simulink model "Coupled_GP_fit"  (R2018b)
settings: Solver=FixedStepAuto  StartTime=0.0  StopTime=t_end  FixedStep=ts  MinStep=1/1e5  RelTol=1e-3
values from neighbouring files (symbols this model uses):
  a0 = omega_n^3    (= 248050213.442)    [TwoLink_init.m]    (also in init.m = 31006276.6803)
  a1 = 3*omega_n^2    (= 1184352.52813)    [TwoLink_init.m]    (also in init.m = 296088.132033)
  a2 = 3*omega_n    (= 1884.95559215)    [TwoLink_init.m]    (also in init.m = 942.477796077)
  b1 = b(:,1)    [init.m]
  b2 = b(:,2)    [init.m]
  D = 50    [Train_SSGP.m]    (also in init.m = 21)
  g = 9.81    [init.m]
  h = 1    [init.m]
  I_limit = 2000    [TwoLink_init.m]
  L1 = 1    [init.m]
  L2 = 1    [init.m]
  m1 = 1    [init.m]
  m2 = 5    [init.m]
  mu_X = mean(xTrain')    [Train_SSGP.m]    (also in init.m = zeros(1,size(n,2)))
  mu_Y = mean(yTrain')    [Train_SSGP.m]    (also in init.m = zeros(1,size(Q,2)))
  N = size(xTrain,2)    [Train_SSGP.m]    (also in init.m = length(noiseSignal))
  r = 5e3    (= 5000)    [init.m]
  R1 = squeeze(R(1,:,:))    [init.m]
  R2 = squeeze(R(2,:,:))    [init.m]
  s = xTrain(:,i_s)'    [Train_SSGP.m]    (also in TwoLink_init.m = tf('s'))
  seed = randi(1e6)    [init.m]
  sf1 = sf(1)    [init.m]
  sf2 = sf(2)    [init.m]
  sig_X = std(xTrain')    [Train_SSGP.m]    (also in init.m = ones(1,size(n,2)))
  sig_Y = std(yTrain')    [Train_SSGP.m]    (also in init.m = ones(1,size(n,2)))
  SIGMA1 = squeeze(SIGMA(1,:,:))    [init.m]
  SIGMA2 = squeeze(SIGMA(2,:,:))    [init.m]
  sp_ts = 2.5    [init.m]
  t_learn = 0    [init.m]
  t_predict = 50    [init.m]
  tm = 2    [init.m]
  ts = 1/1000    (= 0.001)    [Train_SSGP.m]    (also in TwoLink_init.m; init.m)
  w1 = w(:,1)    [init.m]
  w2 = w(:,2)    [init.m]
  X = squeeze(xTraining(:,1,:))'    [init.m]    (also in plot_train_data.m = squeeze(input_vector.Data(:,:,ts_index)))
  Y = yTraining    [init.m]
undefined symbols (not defined in the file or in its folder): DiscIntNeverNeededParam, FF, noise, PID, Z
libraries: sm_lib x13, simulink x6, nesl_utility x5
(part 2 of 2)

== system Coupled_GP_fit/Setpoint Generator/TDfhan1 ==
  V : Inport
  Constant : Constant  Value=r
  Constant1 : Constant  Value=h
  Discrete-Time Integrator : DiscreteIntegrator  gainval=1  SampleTime=ts  ICPrevOutput=DiscIntNeverNeededParam  ICPrevScaledInput=DiscIntNeverNeededParam
  Discrete-Time Integrator1 : DiscreteIntegrator  gainval=1  SampleTime=ts  ICPrevOutput=DiscIntNeverNeededParam  ICPrevScaledInput=DiscIntNeverNeededParam
  MATLAB Function2 : MATLAB Function  TreatAsAtomicUnit=on
  Scope : Scope  NumInputPorts=3
  Sum : Sum  Inputs=+-|
  V1 : Outport
  V2 : Outport  Port=2
  V3 : Outport  Port=3
  wires:
  Discrete-Time Integrator/1 -> Discrete-Time Integrator1/1, MATLAB Function2/2(v2), Scope/2, V2/1  "V2"
  Discrete-Time Integrator1/1 -> Scope/1, V1/1, Sum/1  "V1"
  MATLAB Function2/1(output) -> Scope/3, V3/1, Discrete-Time Integrator/1  "fv"
  Sum/1 -> MATLAB Function2/1(v1)
  V/1 -> Sum/2
  Constant/1 -> MATLAB Function2/3(r0)
  Constant1/1 -> MATLAB Function2/4(h0)

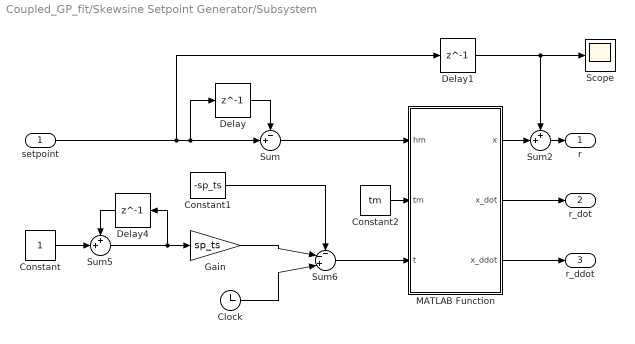
== system Coupled_GP_fit/Skewsine Setpoint Generator/Subsystem ==
  setpoint : Inport
  Clock : Clock
  Constant : Constant  SampleTime=sp_ts
  Constant1 : Constant  Value=-sp_ts  SampleTime=sp_ts
  Constant2 : Constant  Value=tm  SampleTime=sp_ts
  Delay : Delay  DelayLength=1  InitialCondition=0  SampleTime=sp_ts
  Delay1 : Delay  DelayLength=1  InitialCondition=0  SampleTime=sp_ts
  Delay4 : Delay  DelayLength=1  InitialCondition=0  SampleTime=sp_ts
  Gain : Gain  Gain=sp_ts
  MATLAB Function : MATLAB Function  TreatAsAtomicUnit=on
  Scope : Scope
  Sum : Sum  Inputs=-+|
  Sum2 : Sum  Inputs=++|
  Sum5 : Sum  Inputs=++|
  Sum6 : Sum  Inputs=--+|
  r : Outport
  r_dot : Outport  Port=2
  r_ddot : Outport  Port=3
  wires:
  Constant2/1 -> MATLAB Function/2(tm)
  MATLAB Function/1(x) -> Sum2/2
  Delay1/1 -> Scope/1, Sum2/1
  Delay4/1 -> Sum5/1
  Sum/1 -> MATLAB Function/1(hm)
  setpoint/1 -> Delay1/1, Delay/1, Sum/2
  Sum2/1 -> r/1
  Sum5/1 -> Delay4/1, Gain/1
  Constant/1 -> Sum5/2
  MATLAB Function/3(x_ddot) -> r_ddot/1
  Clock/1 -> Sum6/3
  Sum6/1 -> MATLAB Function/3(t)
  Delay/1 -> Sum/1
  Gain/1 -> Sum6/2
  Constant1/1 -> Sum6/1
  MATLAB Function/2(x_dot) -> r_dot/1

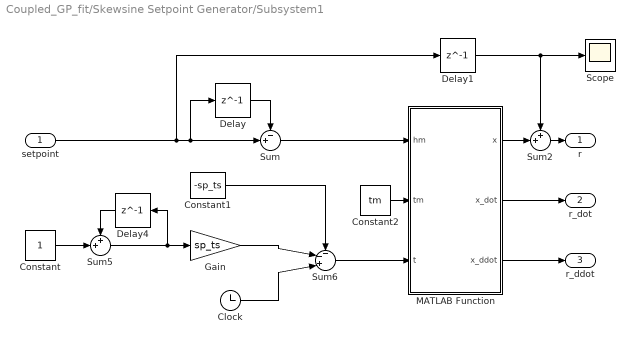
== system Coupled_GP_fit/Skewsine Setpoint Generator/Subsystem1 ==
  setpoint : Inport
  Clock : Clock
  Constant : Constant  SampleTime=sp_ts
  Constant1 : Constant  Value=-sp_ts  SampleTime=sp_ts
  Constant2 : Constant  Value=tm  SampleTime=sp_ts
  Delay : Delay  DelayLength=1  InitialCondition=0  SampleTime=sp_ts
  Delay1 : Delay  DelayLength=1  InitialCondition=0  SampleTime=sp_ts
  Delay4 : Delay  DelayLength=1  InitialCondition=0  SampleTime=sp_ts
  Gain : Gain  Gain=sp_ts
  MATLAB Function : MATLAB Function  TreatAsAtomicUnit=on
  Scope : Scope
  Sum : Sum  Inputs=-+|
  Sum2 : Sum  Inputs=++|
  Sum5 : Sum  Inputs=++|
  Sum6 : Sum  Inputs=--+|
  r : Outport
  r_dot : Outport  Port=2
  r_ddot : Outport  Port=3
  wires:
  Constant2/1 -> MATLAB Function/2(tm)
  MATLAB Function/1(x) -> Sum2/2
  Delay1/1 -> Scope/1, Sum2/1
  Delay4/1 -> Sum5/1
  Sum/1 -> MATLAB Function/1(hm)
  setpoint/1 -> Delay1/1, Delay/1, Sum/2
  Sum2/1 -> r/1
  Sum5/1 -> Delay4/1, Gain/1
  Constant/1 -> Sum5/2
  MATLAB Function/3(x_ddot) -> r_ddot/1
  Clock/1 -> Sum6/3
  Sum6/1 -> MATLAB Function/3(t)
  Delay/1 -> Sum/1
  Gain/1 -> Sum6/2
  Constant1/1 -> Sum6/1
  MATLAB Function/2(x_dot) -> r_dot/1

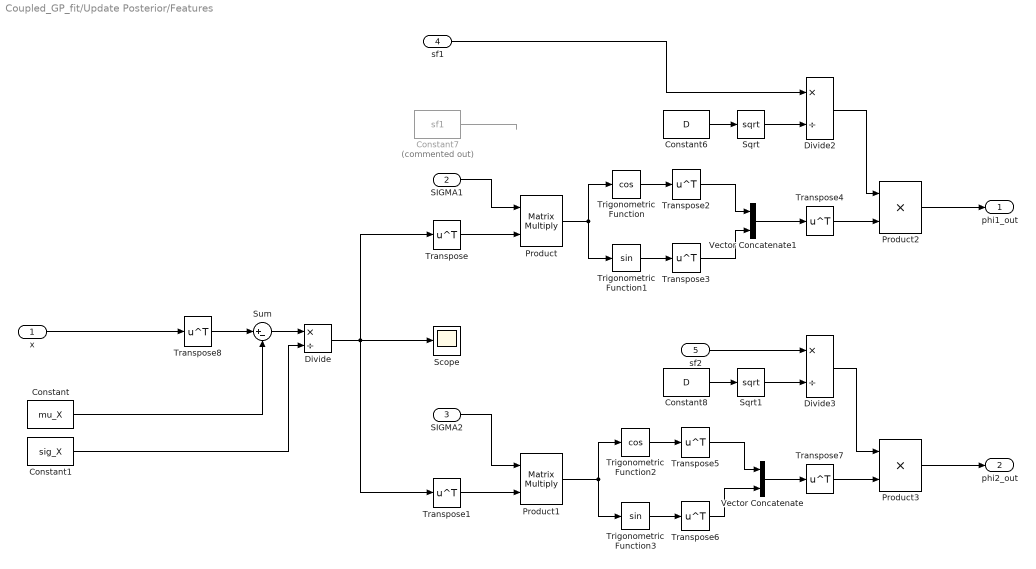
== system Coupled_GP_fit/Update Posterior/Features ==
  x : Inport
  SIGMA1 : Inport  Port=2
  SIGMA2 : Inport  Port=3
  sf1 : Inport  Port=4
  sf2 : Inport  Port=5
  Constant : Constant  Value=mu_X  VectorParams1D=off
  Constant1 : Constant  Value=sig_X  VectorParams1D=off
  Constant6 : Constant  Value=D  SampleTime=-1
  Constant7 : Constant  Commented=on  Value=sf1  SampleTime=-1
  Constant8 : Constant  Value=D  SampleTime=-1
  Divide : Product  Inputs=*/
  Divide2 : Product  Inputs=*/
  Divide3 : Product  Inputs=*/
  Product : Product  Multiplication=Matrix(*)
  Product1 : Product  Multiplication=Matrix(*)
  Product2 : Product
  Product3 : Product
  Scope : Scope
  Sqrt : Sqrt  SaturateOnIntegerOverflow=on
  Sqrt1 : Sqrt  SaturateOnIntegerOverflow=on
  Sum : Sum  Inputs=|+-
  Transpose{,1..8} (9 alike) : Math  Operator=transpose  SaturateOnIntegerOverflow=on
  Trigonometric Function : Trigonometry  Operator=cos
  Trigonometric Function1 : Trigonometry
  Trigonometric Function2 : Trigonometry  Operator=cos
  Trigonometric Function3 : Trigonometry
  Vector Concatenate : Concatenate
  Vector Concatenate1 : Concatenate
  phi1_out : Outport
  phi2_out : Outport  Port=2
  wires:
  Sum/1 -> Divide/1
  Transpose7/1 -> Product3/2
  sf2/1 -> Divide3/1
  SIGMA1/1 -> Product/1
  Transpose1/1 -> Product1/2
  Vector Concatenate/1 -> Transpose7/1
  Product2/1 -> phi1_out/1
  Constant6/1 -> Sqrt/1
  Sqrt1/1 -> Divide3/2
  Trigonometric Function3/1 -> Transpose6/1
  Divide3/1 -> Product3/1
  Trigonometric Function1/1 -> Transpose3/1
  Trigonometric Function/1 -> Transpose2/1
  Constant7/1 -> ?
  Vector Concatenate1/1 -> Transpose4/1
  SIGMA2/1 -> Product1/1
  Transpose3/1 -> Vector Concatenate1/2
  Product/1 -> Trigonometric Function1/1, Trigonometric Function/1
  Constant1/1 -> Divide/2
  Transpose/1 -> Product/2
  Divide/1 -> Scope/1, Transpose/1, Transpose1/1
  Divide2/1 -> Product2/1
  Transpose4/1 -> Product2/2
  Product1/1 -> Trigonometric Function2/1, Trigonometric Function3/1
  Transpose6/1 -> Vector Concatenate/2
  Constant8/1 -> Sqrt1/1
  Trigonometric Function2/1 -> Transpose5/1
  Product3/1 -> phi2_out/1
  Sqrt/1 -> Divide2/2
  Transpose5/1 -> Vector Concatenate/1
  Constant/1 -> Sum/2
  Transpose2/1 -> Vector Concatenate1/1
  x/1 -> Transpose8/1
  Transpose8/1 -> Sum/1
  sf1/1 -> Divide2/1

== matlab function Coupled_GP_fit/Rigid body dynamics/MATLAB Function ==
  settings: updateMethod=DISCRETE  sampleTime=ts
  data: q input size=[2,1]; FF_rgd1 output size=1; q_dot input size=[2,1]; q_ddot input size=[2,1]; q_r_dot input size=[2,1]; q_r_ddot input size=[2,1]; param parameter; FF_rbd2 output size=1
function [FF_rgd1,FF_rbd2] = fcn(q,q_dot,q_ddot,q_r_dot,q_r_ddot,param)
% From: "A Mathematical Introduction to Robotic Manipulation" - Murray

%Model parameters
L1 = param(1);      %[m]  Length link 1
L2 = param(2);      %[m]  Length
r1 = param(3);      %[m]  Length to mass middle point 1
r2 = param(4);      %[m]  Length to mass middle point 2
m1 = param(5);      %[kg] Mass link 1
m2 = param(6);      %[kg] Mass link 2
I1 = param(7);      %[kg.m^2] Moment of inertia link 1
I2 = param(8);      %[kg.m^2] Moment of inertia link 2

alpha = I1+I2+m1*r1^2+m2*(L1^2+r2^2);
beta  = m2*L1*r2;
gamma = I2+m2*r2^2;

c2 = cos(q(2));     %Precalculate cos
s2 = sin(q(2));     %Precalculate sin

M_hat = [alpha+2*beta*c2, gamma+beta*c2;
    gamma+beta*c2, gamma];

C_hat = [-beta*s2*q_dot(2), -beta*s2*(q_dot(1)+q_dot(2));
    beta*s2*q_dot(1), 0];

P_hat = M_hat*q_r_ddot+C_hat*q_r_dot;
FF_rgd1 = P_hat(1);
FF_rbd2 = P_hat(2);

== matlab function Coupled_GP_fit/Update Posterior/MATLAB Function2 ==
  settings: updateMethod=DISCRETE  sampleTime=ts
  data: R_out output; phi input; R1 input
function R_out = cholupdate_fcn(phi,R1)
persistent R; 
if(isempty(R))
    R = R1;
end
R = cholupdate(R,phi);
R_out = R;

== matlab function Coupled_GP_fit/Rigid body dynamics - 2/MATLAB Function ==
  settings: updateMethod=DISCRETE  sampleTime=ts
  data: q input size=[2,1]; T_ff1 output; q_dot input size=[2,1]; q_ddot input size=[2,1]; q_r_dot input size=[2,1]; q_r_ddot input size=[2,1]; param parameter; T_ff2 output
function [T_ff1,T_ff2] = fcn(q,q_dot,q_ddot,q_r_dot,q_r_ddot,param)
L1 = param(1);
L2 = param(2);
r1 = param(3);
r2 = param(4);
m1 = param(5);
m2 = param(6);
I1 = param(7);
I2 = param(8);

alpha = I1+I2+m1*r1^2+m2*(L1^2+r2^2);
beta = m2*L1*r2;
gamma = I2+m2*r2^2;

c2 = cos(q(2));
s2 = sin(q(2));

M_hat = [alpha+2*beta*c2, gamma+beta*c2;
    gamma+beta*c2, gamma];

C_hat = [-beta*s2*q_dot(2), -beta*s2*(q_dot(1)+q_dot(2));
    beta*s2*q_dot(1), 0];

P_hat = M_hat*q_r_ddot+C_hat*q_r_dot;
T_ff1 = P_hat(1);
T_ff2 = P_hat(2);

== matlab function Coupled_GP_fit/Update Posterior/MATLAB Function1 ==
  settings: updateMethod=DISCRETE  sampleTime=ts
  data: R_out output; phi input; R1 input
function R_out = cholupdate_fcn(phi,R1)
persistent R; 
if(isempty(R))
    R = R1;
end
R = cholupdate(R,phi);
R_out = R;

== matlab function Coupled_GP_fit/Update Posterior/MATLAB Function4 ==
  settings: updateMethod=DISCRETE  sampleTime=ts
  data: update input; b_out output; b_init input
function b_out = fcn(update, b_init)
persistent b 
if(isempty(b))
    b = b_init;
end

b = b + update;
b_out = b;

== matlab function Coupled_GP_fit/Update Posterior/MATLAB Function6 ==
  settings: updateMethod=DISCRETE  sampleTime=ts
  data: update input; b_out output; b_init input
function b_out = fcn(update, b_init)
persistent b 
if(isempty(b))
    b = b_init;
end

b = b + update;
b_out = b;

== matlab function Coupled_GP_fit/Setpoint Generator/TDfhan/MATLAB Function2 ==
  data: v1 input; output output; v2 input; r0 input; h0 input
function output = Fhan(v1,v2,r0,h0)
d = h0^2*r0;
a0 = h0*v2;
y = v1 + a0;
a1 = sqrt(d*(d+8*abs(y)));
a2 = a0 + sign(y)*(a1-d)/2;
sy = (sign(y+d)-sign(y-d))/2;
a = (a0+y-a2)*sy +a2;
sa = (sign(a+d)-sign(a-d))/2;
output = -r0 *(a/d -sign(a) )*sa - r0*sign(a);

== matlab function Coupled_GP_fit/Setpoint Generator/TDfhan1/MATLAB Function2 ==
  data: v1 input; output output; v2 input; r0 input; h0 input
function output = Fhan(v1,v2,r0, h0)
d = h0^2*r0;
a0 = h0*v2;
y = v1 + a0;
a1 = sqrt(d*(d+8*abs(y)));
a2 = a0 + sign(y)*(a1-d)/2;
sy = (sign(y+d)-sign(y-d))/2;
a = (a0+y-a2)*sy +a2;
sa = (sign(a+d)-sign(a-d))/2;
output = -r0 *(a/d -sign(a) )*sa - r0*sign(a);

== matlab function Coupled_GP_fit/Skewsine Setpoint Generator/Subsystem1/MATLAB Function ==
  settings: updateMethod=DISCRETE  sampleTime=ts
  data: hm input; x output; tm input; t input; x_dot output; x_ddot output
function [x,x_dot,x_ddot] = skewSine(hm,tm,t)

if (t>=0) && (t<=tm)
    x      = hm/tm*t - hm/(2*pi)*sin(2*pi/tm*t);
    x_dot  = hm/tm - hm/tm*cos(2*pi/tm*t);
    x_ddot = 2*pi*hm/(tm^2)*sin(2*pi/tm*t);
else
    x      = hm;
    x_dot  = 0;
    x_ddot = 0;
end

== matlab function Coupled_GP_fit/Skewsine Setpoint Generator/Subsystem/MATLAB Function ==
  settings: updateMethod=DISCRETE  sampleTime=ts
  data: hm input; x output; tm input; t input; x_dot output; x_ddot output
function [x,x_dot,x_ddot] = skewSine(hm,tm,t)

if (t>=0) && (t<=tm)
    x      = hm/tm*t - hm/(2*pi)*sin(2*pi/tm*t);
    x_dot  = hm/tm - hm/tm*cos(2*pi/tm*t);
    x_ddot = 2*pi*hm/(tm^2)*sin(2*pi/tm*t);
else
    x      = hm;
    x_dot  = 0;
    x_ddot = 0;
end
